simulink model "P4"  (R2020b)
settings: Solver=VariableStepAuto  StartTime=0.0  StopTime=20  RelTol=1e-3
values from neighbouring files (symbols this model uses):
  A1 = 3    [P4_1.m]
  A2 = 5    [P4_1.m]
  g = 9.81    [P2_1.m]    (also in P4_1.m = 32.2)
  h01 = 2    [P4_1.m]
  h02 = 5    [P4_1.m]
  qmi1 = 0.5    [P4_1.m]
  R_L1 = 1E6    (= 1000000)    [P4_1.m]
  R_L2 = 30    [P4_1.m]
  R_R1 = 30    [P4_1.m]
  R_R2 = 40    [P4_1.m]
  rho = 1.94    [P4_1.m]
  timestep1 = 0    [P4_1.m]
settings Model: Creator=mac  LastModifiedBy=li
settings DebuggingCC: SFMachineParentedDataDiag=error

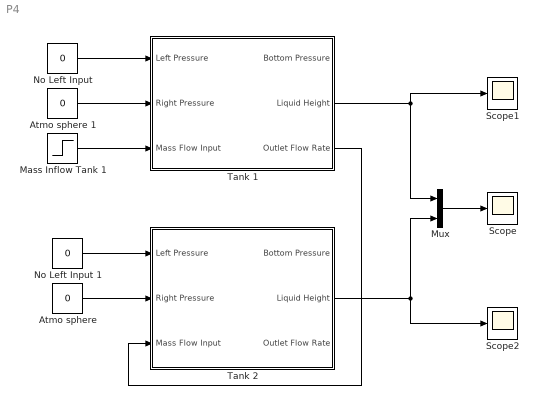
== system P4 ==
  Atmo sphere : Constant  Value=0
  Atmo sphere 1 : Constant  Value=0
  Mass Inflow Tank 1 : Step  Time=timestep1  After=qmi1  SampleTime=0
  Mux : Mux  Inputs=2
  No Left Input : Constant  Value=0
  No Left Input 1 : Constant  Value=0
  Scope : Scope
  Scope1 : Scope
  Scope2 : Scope
  Tank 1 : Subsystem  TreatAsAtomicUnit=on
  Tank 2 : Subsystem  TreatAsAtomicUnit=on
  wires:
  Mass Inflow Tank 1/1 -> Tank 1/3(Mass Flow Input)
  No Left Input/1 -> Tank 1/1(Left Pressure)
  Atmo sphere 1/1 -> Tank 1/2(Right Pressure)
  No Left Input 1/1 -> Tank 2/1(Left Pressure)
  Atmo sphere/1 -> Tank 2/2(Right Pressure)
  Tank 1/3(Outlet Flow Rate) -> Tank 2/3(Mass Flow Input)
  Mux/1 -> Scope/1
  Tank 1/2(Liquid Height) -> Mux/1, Scope1/1
  Tank 2/2(Liquid Height) -> Mux/2, Scope2/1

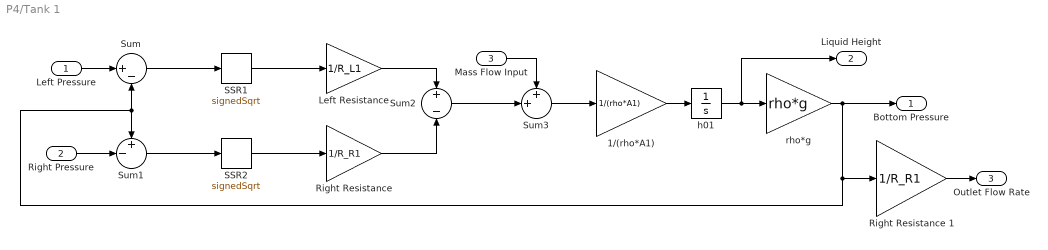
== system P4/Tank 1 ==
  Left Pressure : Inport
  Right Pressure : Inport  Port=2
  Mass Flow Input : Inport  Port=3
  1/(rho*A1) : Gain  Gain=1/(rho*A1)
  Left Resistance : Gain  Gain=1/R_L1
  Right Resistance : Gain  Gain=1/R_R1
  Right Resistance 1 : Gain  Gain=1/R_R1
  SSR1 : Sqrt  Operator=signedSqrt  SaturateOnIntegerOverflow=on
  SSR2 : Sqrt  Operator=signedSqrt  SaturateOnIntegerOverflow=on
  Sum : Sum  Inputs=|+-
  Sum1 : Sum  Inputs=+-|
  Sum2 : Sum  Inputs=+|-
  Sum3 : Sum  Inputs=++|
  h01 : Integrator  InitialCondition=h01
  rho*g : Gain  Gain=rho*g
  Bottom Pressure : Outport  VectorParamsAs1DForOutWhenUnconnected=off
  Liquid Height : Outport  Port=2  VectorParamsAs1DForOutWhenUnconnected=off
  Outlet Flow Rate : Outport  Port=3  VectorParamsAs1DForOutWhenUnconnected=off
  wires:
  1/(rho*A1)/1 -> h01/1
  Right Resistance/1 -> Sum2/2
  h01/1 -> Liquid Height/1, rho*g/1
  Left Resistance/1 -> Sum2/1
  Sum2/1 -> Sum3/2
  Sum3/1 -> 1/(rho*A1)/1
  Left Pressure/1 -> Sum/1
  rho*g/1 -> Sum/2, Sum1/1, Right Resistance 1/1, Bottom Pressure/1
  Mass Flow Input/1 -> Sum3/1
  Right Pressure/1 -> Sum1/2
  Right Resistance 1/1 -> Outlet Flow Rate/1
  Sum1/1 -> SSR2/1
  Sum/1 -> SSR1/1
  SSR1/1 -> Left Resistance/1
  SSR2/1 -> Right Resistance/1

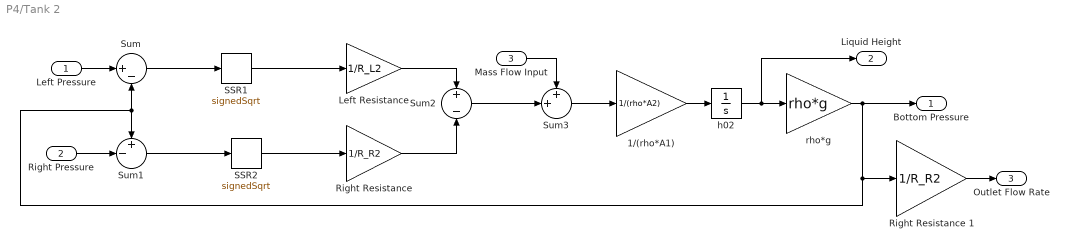
== system P4/Tank 2 ==
  Left Pressure : Inport
  Right Pressure : Inport  Port=2
  Mass Flow Input : Inport  Port=3
  1/(rho*A1) : Gain  Gain=1/(rho*A2)
  Left Resistance : Gain  Gain=1/R_L2
  Right Resistance : Gain  Gain=1/R_R2
  Right Resistance 1 : Gain  Gain=1/R_R2
  SSR1 : Sqrt  Operator=signedSqrt  SaturateOnIntegerOverflow=on
  SSR2 : Sqrt  Operator=signedSqrt  SaturateOnIntegerOverflow=on
  Sum : Sum  Inputs=|+-
  Sum1 : Sum  Inputs=+-|
  Sum2 : Sum  Inputs=+|-
  Sum3 : Sum  Inputs=++|
  h02 : Integrator  InitialCondition=h02
  rho*g : Gain  Gain=rho*g
  Bottom Pressure : Outport  VectorParamsAs1DForOutWhenUnconnected=off
  Liquid Height : Outport  Port=2  VectorParamsAs1DForOutWhenUnconnected=off
  Outlet Flow Rate : Outport  Port=3  VectorParamsAs1DForOutWhenUnconnected=off
  wires:
  Sum2/1 -> Sum3/2
  Right Resistance/1 -> Sum2/2
  Left Resistance/1 -> Sum2/1
  Mass Flow Input/1 -> Sum3/1
  1/(rho*A1)/1 -> h02/1
  h02/1 -> Liquid Height/1, rho*g/1
  Right Pressure/1 -> Sum1/2
  Left Pressure/1 -> Sum/1
  Right Resistance 1/1 -> Outlet Flow Rate/1
  Sum3/1 -> 1/(rho*A1)/1
  rho*g/1 -> Sum/2, Sum1/1, Right Resistance 1/1, Bottom Pressure/1
  Sum/1 -> SSR1/1
  Sum1/1 -> SSR2/1
  SSR1/1 -> Left Resistance/1
  SSR2/1 -> Right Resistance/1
